simulink model "mpc_test"  (R2014a)
settings: Solver=VariableStepDiscrete  StartTime=0.0  StopTime=10.0  RelTol=1e-10
settings Model: Creator=AHMED  LastModifiedBy=AHMED

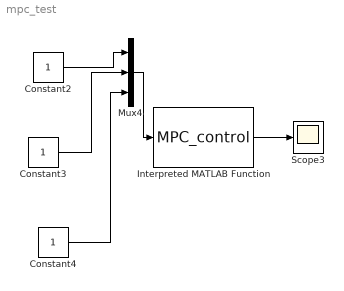
== system mpc_test ==
  Constant2 : Constant  SampleTime=0.001
  Constant3 : Constant  SampleTime=0.001
  Constant4 : Constant  SampleTime=0.001
  Interpreted MATLAB Function : MATLABFcn  MATLABFcn=MPC_control  OutputDimensions=3  SampleTime=0.001
  Mux4 : Mux  Inputs=3
  Scope3 : Scope
      settings: YMin=2.77556e-17  YMax=0.75  SaveName=ScopeData11
  wires:
  Constant2/1 -> Mux4/1
  Constant3/1 -> Mux4/2
  Constant4/1 -> Mux4/3
  Interpreted MATLAB Function/1 -> Scope3/1
  Mux4/1 -> Interpreted MATLAB Function/1
